simulink model "LibraryReference"
settings: configuration reference "?" (kept outside this file)
libraries: AtomicLibrary x10

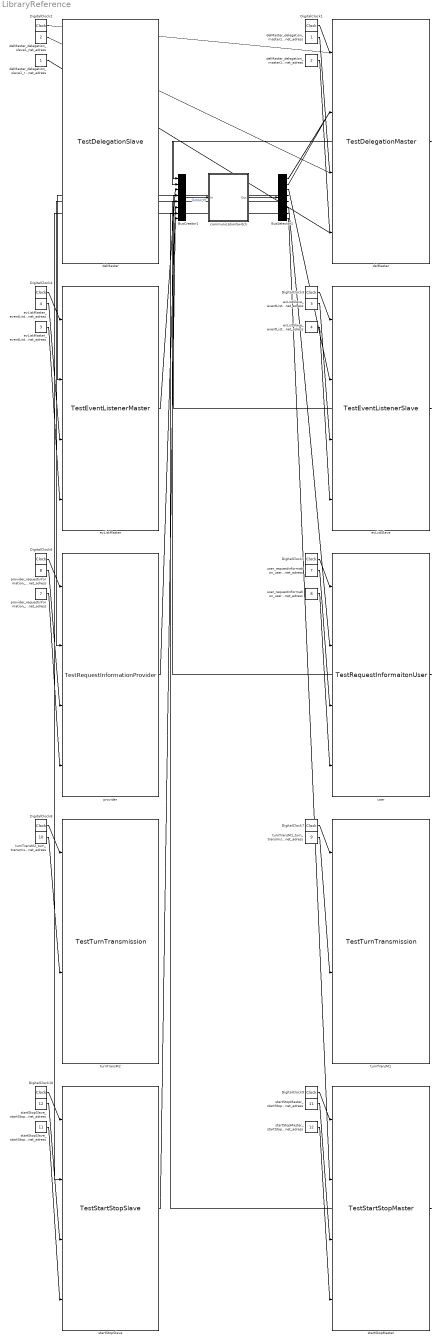
== system LibraryReference ==
  communicationSwitch : Subsystem  Tag=id=_qZ3HAvdmEeGH_6eRdlYQdA
  BusCreator1 : BusCreator  Inputs=8  UseBusObject=on  Tag=id=_qZi98PdmEeGH_6eRdlYQdA
      settings: BusObject=RailCabBus
  BusSelector1 : BusSelector  OutputSignals=Outport1,Outport2,Outport3,Outport4,Outport5,Outport6,Outport7,Outport8  Tag=id=_qZyOgPdmEeGH_6eRdlYQdA
  delMaster : AtomicLibrary/TestDelegationMaster  Tag=id=_qb9YwPdmEeGH_6eRdlYQdA
  DigitalClock1 : DigitalClock  Tag=id=_qcLbMPdmEeGH_6eRdlYQdA  SampleTime=1.0
  delMaster : AtomicLibrary/TestDelegationSlave  Tag=id=_qcSI4PdmEeGH_6eRdlYQdA
  DigitalClock2 : DigitalClock  Tag=id=_qcSv8PdmEeGH_6eRdlYQdA  SampleTime=1.0
  evListSlave : AtomicLibrary/TestEventListenerSlave  Tag=id=_qcb54PdmEeGH_6eRdlYQdA
  DigitalClock3 : DigitalClock  Tag=id=_qcb54fdmEeGH_6eRdlYQdA  SampleTime=1.0
  evListMaster : AtomicLibrary/TestEventListenerMaster  Tag=id=_qclD0PdmEeGH_6eRdlYQdA
  DigitalClock4 : DigitalClock  Tag=id=_qcxREPdmEeGH_6eRdlYQdA  SampleTime=1.0
  user : AtomicLibrary/TestRequestInformaitonUser  Tag=id=_qdebsPdmEeGH_6eRdlYQdA
  DigitalClock5 : DigitalClock  Tag=id=_qdfCwPdmEeGH_6eRdlYQdA  SampleTime=1.0
  provider : AtomicLibrary/TestRequestInformationProvider  Tag=id=_qdykwPdmEeGH_6eRdlYQdA
  DigitalClock6 : DigitalClock  Tag=id=_qdzL0PdmEeGH_6eRdlYQdA  SampleTime=1.0
  turnTransM1 : AtomicLibrary/TestTurnTransmission  Tag=id=_qeCcYPdmEeGH_6eRdlYQdA
  DigitalClock7 : DigitalClock  Tag=id=_qeDDcPdmEeGH_6eRdlYQdA  SampleTime=1.0
  turnTransM2 : AtomicLibrary/TestTurnTransmission  Tag=id=_qeRF4PdmEeGH_6eRdlYQdA
  DigitalClock8 : DigitalClock  Tag=id=_qeRs8PdmEeGH_6eRdlYQdA  SampleTime=1.0
  startStopMaster : AtomicLibrary/TestStartStopMaster  Tag=id=_qeoSQPdmEeGH_6eRdlYQdA
  DigitalClock9 : DigitalClock  Tag=id=_qeo5UPdmEeGH_6eRdlYQdA  SampleTime=1.0
  startStopSlave : AtomicLibrary/TestStartStopSlave  Tag=id=_qe9CYPdmEeGH_6eRdlYQdA
  DigitalClock10 : DigitalClock  Tag=id=_qe9pcPdmEeGH_6eRdlYQdA  SampleTime=1.0
  delMaster_delegation_slave1_net_adress : Constant  Tag=id=_sqGrUPdmEeGH_6eRdlYQdA  Value=2  OutDataType=fixdt(1,16,0)  OutScaling=[]  OutDataTypeStr=Inherit: Inherit from 'Constant value'
  delMaster_delegation_master1_net_adress : Constant  Tag=id=_sqOAEfdmEeGH_6eRdlYQdA  Value=1  OutDataType=fixdt(1,16,0)  OutScaling=[]  OutDataTypeStr=Inherit: Inherit from 'Constant value'
  evListSlave_eventListener_slave1_net_adress : Constant  Tag=id=_sqXxEfdmEeGH_6eRdlYQdA  Value=3  OutDataType=fixdt(1,16,0)  OutScaling=[]  OutDataTypeStr=Inherit: Inherit from 'Constant value'
  evListMaster_eventListener_master1_net_adress : Constant  Tag=id=_sqhiEPdmEeGH_6eRdlYQdA  Value=4  OutDataType=fixdt(1,16,0)  OutScaling=[]  OutDataTypeStr=Inherit: Inherit from 'Constant value'
  turnTransM1_turn_transmission_partner1_net_adress : Constant  Tag=id=_sqqE8fdmEeGH_6eRdlYQdA  Value=9  OutDataType=fixdt(1,16,0)  OutScaling=[]  OutDataTypeStr=Inherit: Inherit from 'Constant value'
  turnTransM2_turn_transmission_partner1_net_adress : Constant  Tag=id=_sqwyofdmEeGH_6eRdlYQdA  Value=10  OutDataType=fixdt(1,16,0)  OutScaling=[]  OutDataTypeStr=Inherit: Inherit from 'Constant value'
  provider_requestinformation_provider1_net_adress : Constant  Tag=id=_sq6jofdmEeGH_6eRdlYQdA  Value=8  OutDataType=fixdt(1,16,0)  OutScaling=[]  OutDataTypeStr=Inherit: Inherit from 'Constant value'
  user_requestinformation_user1_net_adress : Constant  Tag=id=_srGJ0fdmEeGH_6eRdlYQdA  Value=7  OutDataType=fixdt(1,16,0)  OutScaling=[]  OutDataTypeStr=Inherit: Inherit from 'Constant value'
  startStopSlave_startStop_Slave_net_adress : Constant  Tag=id=_srP60fdmEeGH_6eRdlYQdA  Value=12  OutDataType=fixdt(1,16,0)  OutScaling=[]  OutDataTypeStr=Inherit: Inherit from 'Constant value'
  startStopMaster_startStop_Master_net_adress : Constant  Tag=id=_srZr0fdmEeGH_6eRdlYQdA  Value=11  OutDataType=fixdt(1,16,0)  OutScaling=[]  OutDataTypeStr=Inherit: Inherit from 'Constant value'
  delMaster_delegation_master1_receiver_net_adress : Constant  Tag=id=_s2rHtfdmEeGH_6eRdlYQdA  Value=2  OutDataType=fixdt(1,16,0)  OutScaling=[]  OutDataTypeStr=Inherit: Inherit from 'Constant value'
  delMaster_delegation_slave1_receiver_net_adress : Constant  Tag=id=_s2sV0fdmEeGH_6eRdlYQdA  Value=1  OutDataType=fixdt(1,16,0)  OutScaling=[]  OutDataTypeStr=Inherit: Inherit from 'Constant value'
  evListMaster_eventListener_master1_receiver_net_adress : Constant  Tag=id=_s3EwVfdmEeGH_6eRdlYQdA  Value=3  OutDataType=fixdt(1,16,0)  OutScaling=[]  OutDataTypeStr=Inherit: Inherit from 'Constant value'
  evListSlave_eventListener_slave1_receiver_net_adress : Constant  Tag=id=_s3F-cfdmEeGH_6eRdlYQdA  Value=4  OutDataType=fixdt(1,16,0)  OutScaling=[]  OutDataTypeStr=Inherit: Inherit from 'Constant value'
  user_requestinformation_user1_receiver_net_adress : Constant  Tag=id=_s4oPgfdmEeGH_6eRdlYQdA  Value=8  OutDataType=fixdt(1,16,0)  OutScaling=[]  OutDataTypeStr=Inherit: Inherit from 'Constant value'
  provider_requestinformation_provider1_receiver_net_adress : Constant  Tag=id=_s4o2kfdmEeGH_6eRdlYQdA  Value=7  OutDataType=fixdt(1,16,0)  OutScaling=[]  OutDataTypeStr=Inherit: Inherit from 'Constant value'
  startStopMaster_startStop_Master_receiver_net_adress : Constant  Tag=id=_s5UzEfdmEeGH_6eRdlYQdA  Value=12  OutDataType=fixdt(1,16,0)  OutScaling=[]  OutDataTypeStr=Inherit: Inherit from 'Constant value'
  startStopSlave_startStop_Slave_receiver_net_adress : Constant  Tag=id=_s5VaIfdmEeGH_6eRdlYQdA  Value=11  OutDataType=fixdt(1,16,0)  OutScaling=[]  OutDataTypeStr=Inherit: Inherit from 'Constant value'
  wires:
  BusCreator1/1 -> communicationSwitch/1(In)  "Outport9"
  communicationSwitch/1(Out) -> BusSelector1/1
  DigitalClock1/1 -> delMaster/1
  DigitalClock2/1 -> delMaster/1
  DigitalClock3/1 -> evListSlave/1
  DigitalClock4/1 -> evListMaster/1
  DigitalClock5/1 -> user/1
  DigitalClock6/1 -> provider/1
  DigitalClock7/1 -> turnTransM1/1
  DigitalClock8/1 -> turnTransM2/1
  DigitalClock9/1 -> startStopMaster/1
  DigitalClock10/1 -> startStopSlave/1
  delMaster_delegation_slave1_net_adress/1 -> delMaster/3
  delMaster_delegation_master1_net_adress/1 -> delMaster/3
  evListSlave_eventListener_slave1_net_adress/1 -> evListSlave/3
  evListMaster_eventListener_master1_net_adress/1 -> evListMaster/3
  turnTransM1_turn_transmission_partner1_net_adress/1 -> turnTransM1/3
  turnTransM2_turn_transmission_partner1_net_adress/1 -> turnTransM2/3
  provider_requestinformation_provider1_net_adress/1 -> provider/3
  user_requestinformation_user1_net_adress/1 -> user/3
  startStopSlave_startStop_Slave_net_adress/1 -> startStopSlave/3
  startStopMaster_startStop_Master_net_adress/1 -> startStopMaster/3
  delMaster/1 -> BusCreator1/1
  delMaster/1 -> BusCreator1/2
  BusSelector1/1 -> delMaster/2
  BusSelector1/2 -> delMaster/2
  delMaster_delegation_master1_receiver_net_adress/1 -> delMaster/4
  delMaster_delegation_slave1_receiver_net_adress/1 -> delMaster/4
  evListMaster/1 -> BusCreator1/3
  evListSlave/1 -> BusCreator1/4
  BusSelector1/3 -> evListSlave/2
  BusSelector1/4 -> evListMaster/2
  evListMaster_eventListener_master1_receiver_net_adress/1 -> evListMaster/4
  evListSlave_eventListener_slave1_receiver_net_adress/1 -> evListSlave/4
  user/1 -> BusCreator1/5
  provider/1 -> BusCreator1/6
  BusSelector1/5 -> provider/2
  BusSelector1/6 -> user/2
  user_requestinformation_user1_receiver_net_adress/1 -> user/4
  provider_requestinformation_provider1_receiver_net_adress/1 -> provider/4
  startStopMaster/1 -> BusCreator1/7
  startStopSlave/1 -> BusCreator1/8
  BusSelector1/7 -> startStopSlave/2
  BusSelector1/8 -> startStopMaster/2
  startStopMaster_startStop_Master_receiver_net_adress/1 -> startStopMaster/4
  startStopSlave_startStop_Slave_receiver_net_adress/1 -> startStopSlave/4

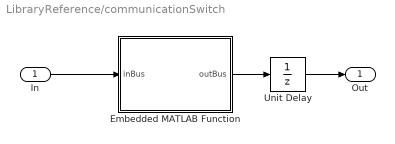
== system LibraryReference/communicationSwitch ==
  In : Inport  Tag=id=_qZ3uEPdmEeGH_6eRdlYQdA  Port=1  PortDimensions=-1  DataType=auto  OutDataType=fixdt(1, 16)  OutScaling=2^0  UseBusObject=on  OutDataTypeStr=Inherit: auto
      settings: BusObject=RailCabBus
  Out : Outport  Tag=id=_qZ4VIPdmEeGH_6eRdlYQdA  Port=1  PortDimensions=-1  DataType=auto  OutDataType=fixdt(1, 16)  OutScaling=2^0  UseBusObject=on  OutDataTypeStr=Inherit: auto
      settings: BusObject=RailCabBus
  Unit Delay : UnitDelay  Tag=id=_qac84PdmEeGH_6eRdlYQdA  SampleTime=-1
  Embedded MATLAB Function : Stateflow chart  Tag=id=_qaNsUPdmEeGH_6eRdlYQdA
  wires:
  In/1 -> Embedded MATLAB Function/1(inBus)
  Unit Delay/1 -> Out/1
  Embedded MATLAB Function/1(outBus) -> Unit Delay/1

== matlab function communicationSwitch/Embedded MATLAB Function ==
  data: inBus input; outBus output
function outBus = BusImpl(inBus)
%#eml
eml.extrinsic('fieldnames','disp','setfield','fprintf');

busSize = numel(inBus.rc1.from);
queueSize = 10*busSize; %length of queue
numShuttles = 0; %Define data type
numShuttles = numel(fieldnames(inBus)); %Shuttles connected to the bus
assert(numShuttles <= 20) %Defines an upper bound for number of shuttles. 
%Important for static memory allocation. 
lookupTableSize = 200;



NOT_ASSIGNED = -1;

%We need persistent queues
persistent queue;
persistent lookupTable;

%Initialize the queues
if isempty(queue)
    queue = repmat(emptyPacket(), numShuttles, queueSize);
end

if isempty(lookupTable)
    lookupTable = repmat(NOT_ASSIGNED, lookupTableSize,1);
end

%Clean outbus
outBus = inBus;
for i = 1:numShuttles
    outBus = setfield(outBus, createRailCabName(i), emptyBus(busSize));
end

%Retrieve packets
for i = 1:numShuttles
    %Get current bus
    currentBus = getBusFromIndex(inBus, busSize, i);
    for j = 1:busSize
        %Read packet
        packet = getPacketFromBus(currentBus, j);
        
        %Check if new packet
        if isValid(packet, numShuttles)
             %Save sender bus element to lookup table
            if lookupTable(packet.from) == NOT_ASSIGNED
                lookupTable(packet.from) = i;
            end
            
            %Save packet in queue
            target = lookupTable(packet.to);
            %Destination unkown. Send to all unassigned.
            if target == NOT_ASSIGNED
                for k = 1:numShuttles
                    if(lookupTable(k) == NOT_ASSIGNED)
                        queue(k,:) = enqueue(queue(k,:), packet); 
                    end
                end                
            %Destination known
            else 
                queue(target,:) = enqueue(queue(target,:), packet);
            end            
        end
    end

end

%Send packet from queue
for i = 1:numShuttles    
    currentBus = getBusFromIndex(outBus, busSize, i);
    for j = 1:busSize
        if ~isEmpty(queue(i,:))
            
            
            %Read last packet
            packet = front(queue(i,:));
            queue(i,:) = dequeue(queue(i,:)); 
            
%            if packet.msg ~= 255 %No ACK
%                fprintf('Sending on port %u[%u/%u]: %s
', i, j, busSize, toString(packet));
%            end            
            
            %Save packet to bus
            currentBus = setPacketToBus(currentBus, j, packet);
            
        else
            break;
        end
    end 
    %Save bus
    outBus = setBusToIndex(outBus, i, currentBus);
end

%%%%%%%%%%%%%%%%%%%%%%%%%%%%%%%%%%%%%%%%%%%%%%%%%%%%%%%%%%%%%%%%%%%%%%%%%%%
%% BUS
%%%%%%%%%%%%%%%%%%%%%%%%%%%%%%%%%%%%%%%%%%%%%%%%%%%%%%%%%%%%%%%%%%%%%%%%%%%

function name = createRailCabName(index) %#eml
%Create name for the railcab used on the bus
eml.extrinsic('sprintf');
name = sprintf('rc%d', index);

function bus = getBusFromIndex(inBus, busSize, index) %eml
%Retrieve a PacketBus from the RailCaBbus
eml.extrinsic('getfield');
busName = createRailCabName(index);
bus = emptyBus(busSize);
bus = getfield(inBus, busName);

function rcBus = setBusToIndex(rcBus, index, packetBus) %eml
%Save a PacketBus to RailCabBus
eml.extrinsic('setfield');
busName = createRailCabName(index);
rcBus = setfield(rcBus, busName, packetBus);

function packet = getPacketFromBus(packetBus, index) %eml
%Retrieve a packet from the bus
packet = emptyPacket();
packet.from = packetBus.from(index);
packet.to = packetBus.to(index);
packet.msg = packetBus.msg(index);
packet.param = packetBus.param (index);
packet.pkgid = packetBus.pkgid(index);
packet.time = packetBus.time(index);

function packetBus = setPacketToBus(packetBus, index, packet) %eml
%Save a packet to the bus
packetBus.from(index) = packet.from;
packetBus.to(index) = packet.to;
packetBus.msg(index) = packet.msg;
packetBus.param (index) = packet.param;
packetBus.pkgid(index) = packet.pkgid;
packetBus.time(index) = packet.time;

function bus = emptyBus(size) %emp
%Create an empty bus
bus = struct('from', zeros(size,1,'uint8'),'to', zeros(size,1,'uint8'),'msg', zeros(size,1,'uint16'),'param', zeros(size,1,'double'),'pkgid', zeros(size,1,'uint32'), 'time', zeros(size,1,'double'));


%%%%%%%%%%%%%%%%%%%%%%%%%%%%%%%%%%%%%%%%%%%%%%%%%%%%%%%%%%%%%%%%%%%%%%%%%%%
%% PACKET
%%%%%%%%%%%%%%%%%%%%%%%%%%%%%%%%%%%%%%%%%%%%%%%%%%%%%%%%%%%%%%%%%%%%%%%%%%%
function packet = emptyPacket() %#eml
%Creates an empty packet
packet = struct('from', uint8(0),'to', uint8(0),'msg', uint16(0),'param', double(0.0),'pkgid', uint32(0), 'time', double(0));

function valid = isValid(packet, numShuttles) %#eml
%Checks wether the given packet is valid and transported by the bus
eml.extrinsic('getfield');
valid = false;
if packet.to > 0 && packet.to <= numShuttles 
    if packet.from > 0 && packet.from <= numShuttles
        valid = true;
    end
end

function packetString = toString(packet) %#eml
eml.extrinsic('sprintf');
packetString = sprintf('%3u: %u->%u :%3u (%.1f) @%.2f', packet.pkgid, packet.from, packet.to, packet.msg, packet.param, packet.time);

%%%%%%%%%%%%%%%%%%%%%%%%%%%%%%%%%%%%%%%%%%%%%%%%%%%%%%%%%%%%%%%%%%%%%%%%%%%
%% QUEUE
%%%%%%%%%%%%%%%%%%%%%%%%%%%%%%%%%%%%%%%%%%%%%%%%%%%%%%%%%%%%%%%%%%%%%%%%%%%

function queue = enqueue(queue, packet) %#eml
%Insert the packet at the end of the queue
eml.extrinsic('warning');
for i=1:length(queue)
    if queue(i).to == 0
        queue(i) = packet;
        return;
    end
end
%No empty entry found
warning('RailCab:Bus','Bus: buffer overflow for outgoing queue to %d', queue(1).to);

function queue = dequeue(queue) %#eml
%Removes the first packet of the queue
for i = 1:length(queue)-1
    queue(i) = queue(i+1);
    if queue(i).to == 0
        %end reached
        return;
    end
end
queue(length(queue)) = emptyPacket();

function packet = front(queue) %#eml
%Returns the first element from the queue
packet = queue(1);

function empty = isEmpty(queue) %#eml
%Checks whether the queue is empty or not
packet = queue(1);
if packet.to == 0
    empty = true;
else
    empty = false;
end
